simulink model "sim_topic3"  (R2023b)
settings: Solver=FixedStepAuto  StartTime=0.0  StopTime=T_sim  FixedStep=dt_sim  RelTol=1e-3
undefined symbols (not defined in the file): Gp_ss, K, T, x0
settings Model: Creator=user  LastModifiedBy=user

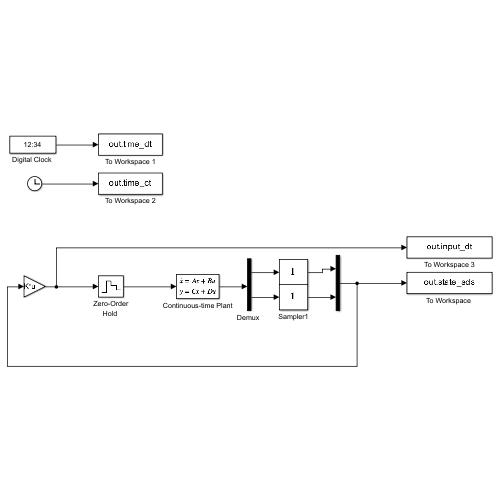
[thumbnail: Simulink's stored preview of the top-level diagram]
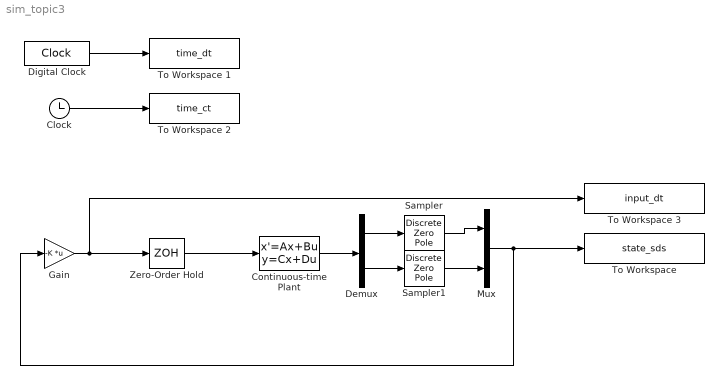
== system sim_topic3 ==
  Clock : Clock
  Continuous-time Plant : StateSpace  A=Gp_ss.A  B=Gp_ss.B  C=eye(2)  D=zeros(2,1)  InitialCondition=x0
  "Demux " : Demux  Outputs=2
  "Digital Clock " : DigitalClock  SampleTime=T
  Gain : Gain  Gain=-K  Multiplication=Matrix(K*u)
  Mux : Mux  Inputs=2
  Sampler : DiscreteZeroPole  Zeros=[]  Poles=[]  Gain=1  SampleTime=T
  Sampler1 : DiscreteZeroPole  Zeros=[]  Poles=[]  Gain=1  SampleTime=T
  "To Workspace " : ToWorkspace  VariableName=state_sds  SampleTime=T
  To Workspace 1 : ToWorkspace  VariableName=time_dt  SampleTime=T
  To Workspace 2 : ToWorkspace  VariableName=time_ct  SampleTime=-1
  To Workspace 3 : ToWorkspace  VariableName=input_dt  SampleTime=T
  "Zero-Order Hold " : ZeroOrderHold  SampleTime=-1
  wires:
  Clock/1 -> To Workspace 2/1
  "Digital Clock "/1 -> To Workspace 1/1
  Gain/1 -> To Workspace 3/1, "Zero-Order Hold "/1
  "Zero-Order Hold "/1 -> Continuous-time Plant/1
  Continuous-time Plant/1 -> "Demux "/1
  "Demux "/1 -> Sampler/1
  "Demux "/2 -> Sampler1/1
  Sampler/1 -> Mux/1
  Sampler1/1 -> Mux/2
  Mux/1 -> "To Workspace "/1, Gain/1
